simulink model "TrayectoriaStateFlowO"  (R2023b)
settings: Solver=VariableStepAuto  StartTime=0.0  StopTime=10.0  RelTol=1e-3
undefined symbols (not defined in the file): d, DiscIntNeverNeededParam
libraries: slpidlib x1
settings Model: Creator=keanu  LastModifiedBy=keanu

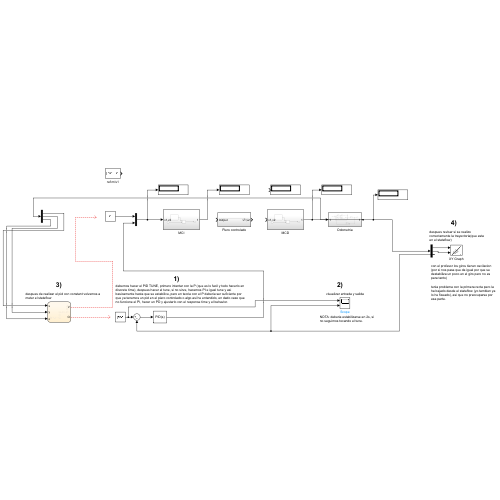
[thumbnail: Simulink's stored preview of the top-level diagram]
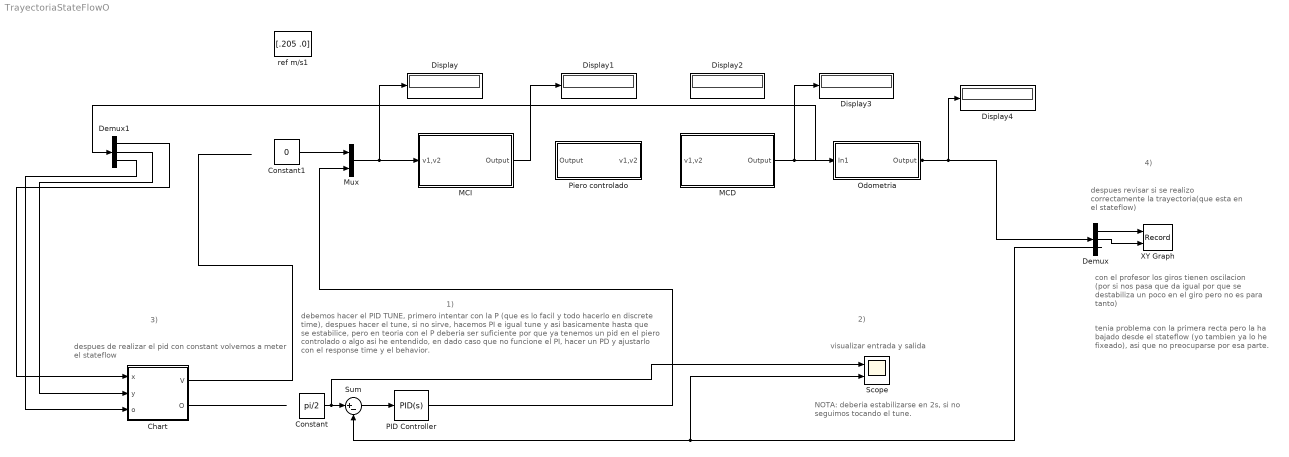
== system TrayectoriaStateFlowO ==
  note: tenia problema con la primera recta pero la ha bajado desde el stateflow (yo tambien ya lo he fixeado), asi que no preocuparse por esa parte.
  note: con el profesor los giros tienen oscilacion (por si nos pasa que da igual por que se destabiliza un poco en el giro pero no es para tanto)
  note: despues revisar si se realizo correctamente la trayectoria(que esta en el stateflow)
  note: 2)
  note: 1)
  note: despues de realizar el pid con constant volvemos a meter el stateflow
  note: NOTA: deberia estabilizarse en 2s, si no seguimos tocando el tune.
  note: visualizar entrada y salida
  note: debemos hacer el PID TUNE, primero intentar con la P (que es lo facil y todo hacerlo en discrete time), despues hacer el tune, si no sirve, hacemos PI e igual tune y asi basicamente hasta que se estabilice, pero en teoria con el P deberia ser suficiente por que ya tenemos un pid en el piero controlado o algo asi he entendido, en dado caso que no funcione el PI, hacer un PD y ajustarlo con el response time y el behavior.
  note: 3)
  note: 4)
  Chart : Stateflow chart  TreatAsAtomicUnit=on
  Constant : Constant  Value=pi/2
  Constant1 : Constant  Value=0
  Demux : Demux  Outputs=3
  Demux1 : Demux  Outputs=3
  Display{,1..4} (5 alike) : Display
  MCD : Subsystem
  MCI : Subsystem
  Mux : Mux  Inputs=2
  Odometria : Subsystem
  PID Controller : slpidlib/PID Controller  Controller=PID  Form=Parallel  TimeDomain=Continuous-time  UseExternalTs=off  SampleTime=-1  IntegratorMethod=Forward Euler  FilterMethod=Forward Euler  ControllerParametersSource=internal  P=1  I=1  UseKiTs=off  D=0  N=100  UseFilter=on  TunerSelectOption=Transfer Function Based (PID Tuner App)  InitialConditionSource=internal  InitialConditionForIntegrator=0  InitialConditionForFilter=0  DifferentiatorICPrevScaledInput=0  ExternalReset=none  TrackingMode=off  Kt=1  LimitOutput=off  SatLimitsSource=internal  UpperSaturationLimit=inf  LowerSaturationLimit=-inf  LinearizeAsGain=on  AntiWindupMode=none  Kb=1  LimitIntegrator=off  UpperIntegratorSaturationLimit=inf  LowerIntegratorSaturationLimit=-inf  POutMin=[]  POutMax=[]  IOutMin=[]  IOutMax=[]  DOutMin=[]  DOutMax=[]  NOutMin=[]  NOutMax=[]  SumOutMin=[]  SumOutMax=[]  SaturationOutMin=[]  SaturationOutMax=[]  PParamMin=[]  PParamMax=[]  IParamMin=[]  IParamMax=[]  DParamMin=[]  DParamMax=[]  NParamMin=[]  NParamMax=[]  KbParamMin=[]  KbParamMax=[]  KtParamMin=[]  KtParamMax=[]  KbOutMin=[]  KbOutMax=[]  KtOutMin=[]  KtOutMax=[]  IntegratorOutMin=[]  IntegratorOutMax=[]  FilterOutMin=[]  FilterOutMax=[]  SumI1OutMin=[]  SumI1OutMax=[]  SumI2OutMin=[]  SumI2OutMax=[]  SumI3OutMin=[]  SumI3OutMax=[]  SumI4OutMin=[]  SumI4OutMax=[]  SumDOutMin=[]  SumDOutMax=[]  DifferentiatorOutMin=[]  DifferentiatorOutMax=[]  FilterDiffOutCoefMin=[]  FilterDiffOutCoefMax=[]  ReciprocalOutMin=[]  ReciprocalOutMax=[]  SumDenOutMin=[]  SumDenOutMax=[]  SumNumOutMin=[]  SumNumOutMax=[]  DivideOutMin=[]  DivideOutMax=[]  UdiffTsProdOutMin=[]  UdiffTsProdOutMax=[]  NTsProdOutMin=[]  NTsProdOutMax=[]  UintegralTsProdOutMin=[]  UintegralTsProdOutMax=[]  UngainTsProdOutMin=[]  UngainTsProdOutMax=[]  ClampingZeroOutDataTypeStr=Inherit: Inherit via back propagation  ClampingZeroOutMin=[]  ClampingZeroOutMax=[]  FilterDenConstantOutDataTypeStr=Inherit: Inherit via back propagation  FilterDenConstantOutMin=[]  FilterDenConstantOutMax=[]  PCopyOutDataTypeStr=Inherit: Inherit via back propagation  PCopyOutMin=[]  PCopyOutMax=[]  NCopyOutDataTypeStr=Inherit: Inherit via back propagation  NCopyOutMin=[]  NCopyOutMax=[]  IntegratorContinuousStateAttributes=''  IntegratorStateMustResolveToSignalObject=off  IntegratorRTWStateStorageClass=Auto  FilterContinuousStateAttributes=''  FilterStateMustResolveToSignalObject=off  FilterRTWStateStorageClass=Auto  ParallelPVariant=InternalParameters  IdealPVariant=Disabled  IVariant=InternalParameters  DVariant=InternalParameters  IntegratorVariant=Continuous  SatVariant=Disabled  AWVariant=Passthrough  PCopyVariant=Disabled  TRVariant=Disabled  FdbkBlocksVariant=Forward  IdealPFdbkVariant=Disabled  SatFdbkVariant=Disabled  DerivativeFilterVariant=ContFilter  NVariant=InternalParameters  NCopyVariant=Disabled  FilterICVariant=InternalICsFilter  IntegratorICVariant=InternalICs  ExternalResetVariant=Disabled  TRSumVariant=Passthrough  SumFdbkVariant=Disabled  SumVariant=Sum_PID  TsampFilterVariant=InternalTs  TsampNgainVariant=Passthrough  TsampIntegralVariant=Passthrough  ExternalSaturationOutDataTypeStr=Inherit: Same as second input
  Piero controlado : Subsystem
  Scope : Scope  NumInputPorts=2
  Sum : Sum  Inputs=|+-
  XY Graph : Record  FileSettingsInternal="{\"entries\":[{\"content\":{\"excelSettings\":{\"content\":{},\"type\":\"Streamout.ExcelSettings\"}},\"type\":\"Streamout.FileSettingStorage\",\"uuid\":\"\"}],\"packageUris\":[\"http:\\/\\/schema.mathworks.com\\/mf0\\/streamout_blocks\\/R2020a\"],\"version\":\"1.0\"}"  Layout=[1 1]  SignalsInternal="{\"entries\":[{\"content\":{\"signals\":[{\"content\":{\"blockPath\":[],\"dimensions\":[1],\"domain\":\"\",\"lineColor\":\"#7e2f8e\",\"port\":1,\"signalID\":1,\"signalName\":\"Demux:1\"},\"type\":\"RecordBlkView.Signal\",\"uuid\":\"\"},{\"content\":{\"blockPath\":[],\"dimensions\":[1],\"domain\":\"\",\"lineColor\":\"#77ac30\",\"port\":2,\"signalID\":2,\"signalName\":\"Demux:2\"},\"type\":\"RecordBlkView.Signal\",\"uuid\":\"\"}]},\"type\":\"RecordBlkView.InputSignals\",\"uuid\":\"\"}],\"packageUris\":[\"http:\\/\\/schema.mathworks.com\\/mf0\\/streamout_blocks\\/R2020a\"],\"version\":\"1.0\"}"  VisualizationBindings="{\"xyplotplugin\":{\"info\":[{\"series\":[],\"subplotID\":1}]}}"  CompatibilityTag=XY
  ref m/s1 : Constant  Value=[.205 .0]
  wires:
  MCD/1(Output) -> Display3/1, Odometria/1(In1)
  Mux/1 -> Display/1, MCI/1(v1,v2)
  MCI/1(Output) -> Display1/1
  Odometria/1(Output) -> Display4/1, Demux/1, Demux1/1
  Demux/1 -> XY Graph/1
  Demux/2 -> XY Graph/2
  Demux1/1 -> Chart/1(x)
  Demux1/2 -> Chart/2(y)
  Demux1/3 -> Chart/3(o)
  Sum/1 -> PID Controller/1
  PID Controller/1 -> Mux/2
  Demux/3 -> Scope/2, Sum/2
  Constant1/1 -> Mux/1
  Constant/1 -> Scope/1, Sum/1
  Chart/1(V) -> ?
  Chart/2(O) -> ?

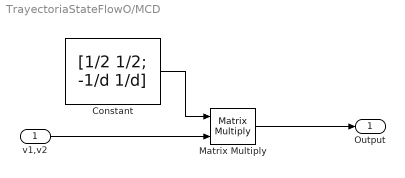
== system TrayectoriaStateFlowO/MCD ==
  v1,v2 : Inport
  Constant : Constant  Value=[1/2 1/2; -1/d 1/d]
  Matrix Multiply : Product  Multiplication=Matrix(*)
  Output : Outport
  wires:
  Matrix Multiply/1 -> Output/1
  v1,v2/1 -> Matrix Multiply/2
  Constant/1 -> Matrix Multiply/1

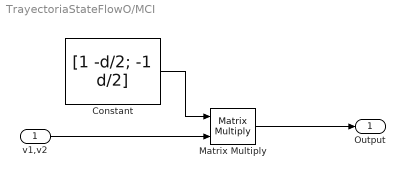
== system TrayectoriaStateFlowO/MCI ==
  v1,v2 : Inport
  Constant : Constant  Value=[1 -d/2; -1 d/2]
  Matrix Multiply : Product  Multiplication=Matrix(*)
  Output : Outport
  wires:
  Constant/1 -> Matrix Multiply/1
  v1,v2/1 -> Matrix Multiply/2
  Matrix Multiply/1 -> Output/1

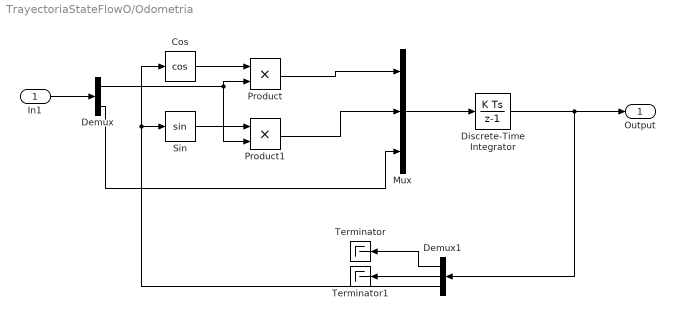
== system TrayectoriaStateFlowO/Odometria ==
  In1 : Inport
  Cos : Trigonometry  Operator=cos
  Demux : Demux  Outputs=2
  Demux1 : Demux  Outputs=3
  Discrete-Time Integrator : DiscreteIntegrator  SampleTime=-1  ICPrevOutput=DiscIntNeverNeededParam  ICPrevScaledInput=DiscIntNeverNeededParam
  Mux : Mux  Inputs=3
  Product : Product
  Product1 : Product
  Sin : Trigonometry
  Terminator : Terminator
  Terminator1 : Terminator
  Output : Outport
  wires:
  Discrete-Time Integrator/1 -> Demux1/1, Output/1
  Product1/1 -> Mux/2
  In1/1 -> Demux/1
  Cos/1 -> Product/1
  Demux/2 -> Mux/3
  Demux1/3 -> Sin/1, Cos/1
  Product/1 -> Mux/1
  Demux1/2 -> Terminator1/1
  Sin/1 -> Product1/1
  Mux/1 -> Discrete-Time Integrator/1
  Demux/1 -> Product1/2, Product/2
  Demux1/1 -> Terminator/1

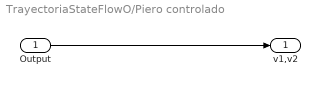
== system TrayectoriaStateFlowO/Piero controlado ==
  Output : Inport
  v1,v2 : Outport
  wires:
  Output/1 -> v1,v2/1

== stateflow chart TrayectoriaStateFlowO/Chart ==
  state Paro
    V=0;
    O=pi/2;
  state Recto2
    V=0.205;
    O=pi/2;
  state GiroDcha
    V=0.10;
    O=0;
  state Recto1
    V=0.205;
    O=0;
  state GiroIzq1
    V=0.10;
    O=pi/2;
  state Recto
    V=0.205;
    O=pi/2;
  state Inicio
    V=0;
    O=0;
    w=0;
  state Marcha
    V=0.205;
    O=0;
  state GiroIzq
    V=0.10;
    O=pi/2;
  Recto2 -> Paro : [y>14]
  GiroIzq1 -> Recto2 : [o>pi/2]
  Recto1 -> GiroIzq1 : [x>3]
  GiroDcha -> Recto1 : [o>0]
  Recto -> GiroDcha : [y>12]
  GiroIzq -> Recto : [o>pi/2]
  (default) -> Inicio
  Inicio -> Marcha : [after(1,sec)]
  Marcha -> GiroIzq : [x>1.7]
  data: V output double size=1; x input double size=1; y input double size=1; o input double size=1; O output
